simulink model "testsingola"  (R2021a)
settings: Solver=VariableStepAuto  StartTime=0.0  StopTime=1000  RelTol=1e-3
values from neighbouring files (symbols this model uses):
  a1 = 0.45    [Malware1.m]    (also in Malware3.m; PLC1.m; PLC3.m; init.m)
  A1 = 154    [Malware1.m]    (also in PLC1.m; init.m)
  a2 = 0.25    [init.m]
  A3 = 154    [Malware3.m]    (also in PLC3.m; init.m)
  g = 980.665    [Malware1.m]    (also in Malware3.m; PLC1.m; PLC3.m; init.m)
  H1_max = 100    [Malware1.m]    (also in PLC1.m; init.m)
  Q1_max = 100    [Malware1.m]    (also in PLC1.m; init.m)
  Q3_max = 10    [Malware3.m]    (also in PLC3.m; init.m)
  s12 = 0.5    [Malware1.m]    (also in Malware3.m; PLC1.m; PLC3.m; init.m)
  s23 = s12    (= 0.5)    [init.m]
libraries: dspnetwork x8
settings Model: Creator=Dottorandi  LastModifiedBy=labo
settings SolverCC: AlgebraicLoopSolver=TrustRegion
settings DataIOCC: ReturnWorkspaceOutputs=off
settings DebuggingCC: SFMachineParentedDataDiag=warning  ArithmeticOperatorsInVariantConditions=warning
settings SFSimCC: SimUseLocalCustomCode=off  CustomCodeUndefinedFunction=UseInterfaceOnly
settings RTWCC: RTWUseLocalCustomCode=off

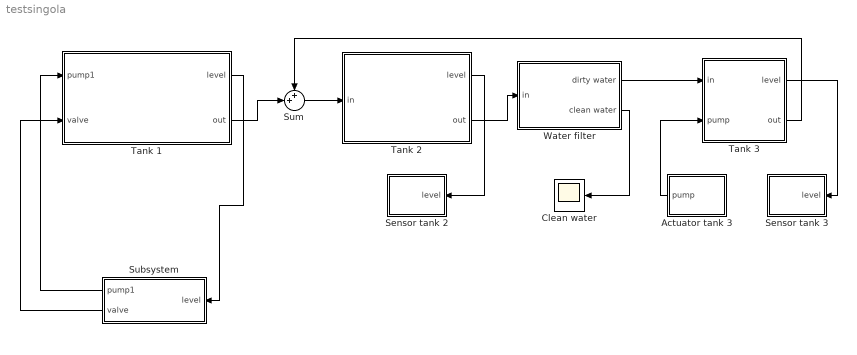
== system testsingola ==
  Actuator tank 3 : Subsystem
  "Clean water " : Scope
  Sensor tank 2 : Subsystem
  Sensor tank 3 : Subsystem
  Subsystem : Subsystem
  Sum : Sum  Inputs=++|
  Tank 1 : Subsystem
  Tank 2 : Subsystem
  Tank 3 : Subsystem
  Water filter : Subsystem
  wires:
  Sum/1 -> Tank 2/1(in)
  Tank 3/2(out) -> Sum/1
  Water filter/2("clean water ") -> "Clean water "/1
  Tank 1/2(out) -> Sum/2
  Tank 2/2(out) -> Water filter/1(in)
  Water filter/1(dirty water) -> Tank 3/1(in)
  Tank 1/1(level) -> Subsystem/1(level)
  Subsystem/1(pump1) -> Tank 1/1(pump1)
  Subsystem/2(valve) -> Tank 1/2(valve)
  Tank 2/1(level) -> Sensor tank 2/1(level)
  Tank 3/1(level) -> Sensor tank 3/1(level)
  Actuator tank 3/1(pump) -> Tank 3/2(pump)

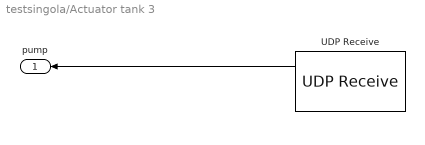
== system testsingola/Actuator tank 3 ==
  UDP Receive : dspnetwork/UDP Receive  localURL='0.0.0.0'  localPort=10003  remoteURL='0.0.0.0'  remotePort=-1  recvBufferSize=2  dims=1  signalDatatype=uint16  isComplex=off  isVarSize=off  showBlockingTime=on  blockingTime=0  sampletime=1  blockPlatform=LINUX
  pump : Outport  VectorParamsAs1DForOutWhenUnconnected=off
  wires:
  UDP Receive/1 -> pump/1

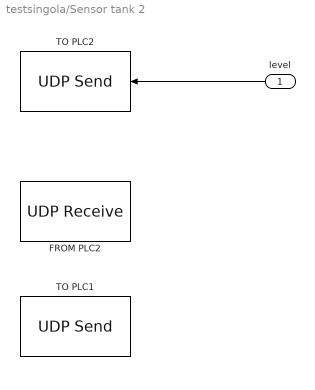
== system testsingola/Sensor tank 2 ==
  level : Inport
  FROM PLC2 : dspnetwork/UDP Receive  localURL='0.0.0.0'  localPort=10003  remoteURL='0.0.0.0'  remotePort=-1  recvBufferSize=2  dims=1  signalDatatype=uint16  isComplex=off  isVarSize=off  showBlockingTime=on  blockingTime=0  sampletime=1  blockPlatform=LINUX
  TO PLC1 : dspnetwork/UDP Send  remoteURL='localhost'  remotePort=10001  localURL='255.255.255.255'  localPortSource=Automatically determine  localPort=-1  sendBufferSize=8192  sampletime=-1  blockPlatform=LINUX  separateLengthPort=0
  TO PLC2 : dspnetwork/UDP Send  remoteURL='localhost'  remotePort=10001  localURL='255.255.255.255'  localPortSource=Automatically determine  localPort=-1  sendBufferSize=8192  sampletime=-1  blockPlatform=LINUX  separateLengthPort=0
  wires:
  level/1 -> TO PLC2/1

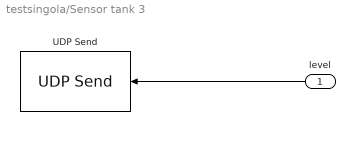
== system testsingola/Sensor tank 3 ==
  level : Inport
  UDP Send : dspnetwork/UDP Send  remoteURL='localhost'  remotePort=10001  localURL='255.255.255.255'  localPortSource=Automatically determine  localPort=-1  sendBufferSize=8192  sampletime=-1  blockPlatform=LINUX  separateLengthPort=0
  wires:
  level/1 -> UDP Send/1

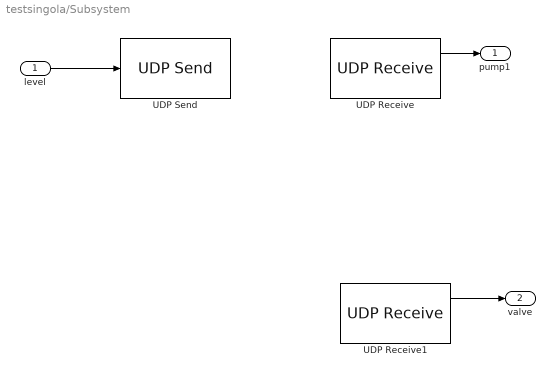
== system testsingola/Subsystem ==
  level : Inport
  UDP Receive : dspnetwork/UDP Receive  localURL='0.0.0.0'  localPort=10002  remoteURL='0.0.0.0'  remotePort=-1  recvBufferSize=2  dims=1  signalDatatype=uint16  isComplex=off  isVarSize=off  showBlockingTime=on  blockingTime=0  sampletime=1  blockPlatform=LINUX
  UDP Receive1 : dspnetwork/UDP Receive  localURL='0.0.0.0'  localPort=10003  remoteURL='0.0.0.0'  remotePort=-1  recvBufferSize=2  dims=1  signalDatatype=uint16  isComplex=off  isVarSize=off  showBlockingTime=on  blockingTime=0  sampletime=1  blockPlatform=LINUX
  UDP Send : dspnetwork/UDP Send  remoteURL='localhost'  remotePort=10001  localURL='255.255.255.255'  localPortSource=Automatically determine  localPort=-1  sendBufferSize=8192  sampletime=-1  blockPlatform=LINUX  separateLengthPort=0
  pump1 : Outport  VectorParamsAs1DForOutWhenUnconnected=off
  valve : Outport  Port=2  VectorParamsAs1DForOutWhenUnconnected=off
  wires:
  level/1 -> UDP Send/1
  UDP Receive/1 -> pump1/1
  UDP Receive1/1 -> valve/1

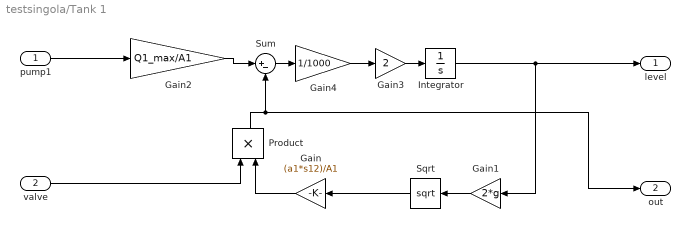
== system testsingola/Tank 1 ==
  pump1 : Inport
  valve : Inport  Port=2
  Gain : Gain  Gain=(a1*s12)/A1
  Gain1 : Gain  Gain=2*g
  Gain2 : Gain  Gain=Q1_max/A1
  Gain3 : Gain  Gain=2
  Gain4 : Gain  Gain=1/1000
  Integrator : Integrator  InitialCondition=0.11*H1_max
  Product : Product
  Sqrt : Sqrt  SaturateOnIntegerOverflow=on
  Sum : Sum  Inputs=|+-
  level : Outport  VectorParamsAs1DForOutWhenUnconnected=off
  out : Outport  Port=2  VectorParamsAs1DForOutWhenUnconnected=off
  wires:
  Integrator/1 -> Gain1/1, level/1
  Sum/1 -> Gain4/1
  Gain/1 -> Product/2
  Sqrt/1 -> Gain/1
  Gain1/1 -> Sqrt/1
  valve/1 -> Product/1
  Product/1 -> out/1, Sum/2
  Gain2/1 -> Sum/1
  pump1/1 -> Gain2/1
  Gain3/1 -> Integrator/1
  Gain4/1 -> Gain3/1

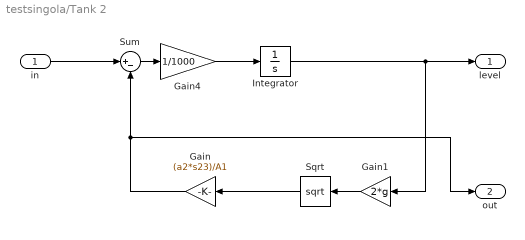
== system testsingola/Tank 2 ==
  in : Inport
  Gain : Gain  Gain=(a2*s23)/A1
  Gain1 : Gain  Gain=2*g
  Gain4 : Gain  Gain=1/1000
  Integrator : Integrator  InitialCondition=0.11*H1_max
  Sqrt : Sqrt  SaturateOnIntegerOverflow=on
  Sum : Sum  Inputs=|+-
  level : Outport  VectorParamsAs1DForOutWhenUnconnected=off
  out : Outport  Port=2  VectorParamsAs1DForOutWhenUnconnected=off
  wires:
  in/1 -> Sum/1
  Integrator/1 -> Gain1/1, level/1
  Sum/1 -> Gain4/1
  Sqrt/1 -> Gain/1
  Gain1/1 -> Sqrt/1
  Gain/1 -> out/1, Sum/2
  Gain4/1 -> Integrator/1

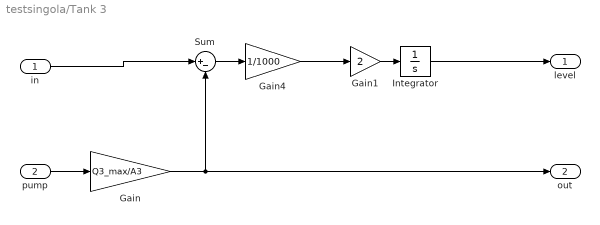
== system testsingola/Tank 3 ==
  in : Inport
  pump : Inport  Port=2
  Gain : Gain  Gain=Q3_max/A3
  Gain1 : Gain  Gain=2
  Gain4 : Gain  Gain=1/1000
  Integrator : Integrator
  Sum : Sum  Inputs=|+-
  level : Outport  VectorParamsAs1DForOutWhenUnconnected=off
  out : Outport  Port=2  VectorParamsAs1DForOutWhenUnconnected=off
  wires:
  Integrator/1 -> level/1
  Sum/1 -> Gain4/1
  pump/1 -> Gain/1
  in/1 -> Sum/1
  Gain/1 -> Sum/2, out/1
  Gain1/1 -> Integrator/1
  Gain4/1 -> Gain1/1

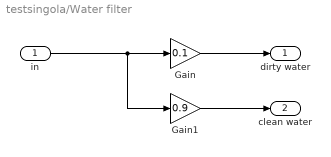
== system testsingola/Water filter ==
  in : Inport
  Gain : Gain  Gain=0.1
  Gain1 : Gain  Gain=0.9
  dirty water : Outport  VectorParamsAs1DForOutWhenUnconnected=off
  "clean water " : Outport  Port=2  VectorParamsAs1DForOutWhenUnconnected=off
  wires:
  in/1 -> Gain1/1, Gain/1
  Gain/1 -> dirty water/1
  Gain1/1 -> "clean water "/1
